simulink model "lss_online"  (R2022b)
settings: Solver=FixedStepAuto  StartTime=0.0  StopTime=Inf  FixedStep=0.001  RelTol=1e-3  EnableMultiTasking=on
InitFcn:
  | clear mex
model workspace (MAT data in the model file):
  worldsim_instance.endpoint_ip = '127.0.0.1'
  worldsim_instance.endpoint_port = 8080
values from neighbouring files (symbols this model uses):
  ADAS_Control_Mode = 1    [LSS_parameters.m]    (also in lss_ini_param.sldd = 1.0)
  AP_Transition_Rate = 0.5    [LSS_parameters.m]    (also in lss_ini_param.sldd = 0.8)
  butter_a = 1.0 -1.9911142922016536 0.99115359586893548    [lss_ini_param.sldd]
  butter_a_lka_out = 1.0 -1.5610180758007179 0.641351538057563    [lss_ini_param.sldd]
  butter_b = 9.825916820482009E-6 1.9651833640964018E-5 9.825916820482009E-6    [lss_ini_param.sldd]
  butter_b_lka_out = 0.020083365564211246 0.040166731128422492 0.020083365564211246    [lss_ini_param.sldd]
  index_variant_approaching_speed = 3.0    [lss_ini_param.sldd]
  LDW_Activity_Flag = 1    [LSS_parameters.m]    (also in lss_ini_param.sldd = 1.0)
  LDW_Freq_Hz = Sensor_Freq_worldsim    [LSS_parameters.m]    (also in lss_ini_param.sldd = 50.0)
  LDW_LaneGap_dydt_Warning = 50    [LSS_parameters.m]    (also in lss_ini_param.sldd = 50.0)
  LDW_LaneGap_Warning = [0.5 0.25]    [LSS_parameters.m]    (also in lss_ini_param.sldd = 0.5 0.25)
  LDW_Min_Speed = 60    [LSS_parameters.m]    (also in lss_ini_param.sldd = 60.0)
  LDW_Steer_Vibration_Amplitude = 5    [LSS_parameters.m]    (also in lss_ini_param.sldd = 5.0)
  LDW_Steer_Vibration_Freq = 25    [LSS_parameters.m]    (also in lss_ini_param.sldd = 25.0)
  LKA_Activity_Flag = 1    [LSS_parameters.m]    (also in lss_ini_param.sldd = 1.0)
  LKA_D = [0.2 0.3]    [LSS_parameters.m]    (also in lss_ini_param.sldd = 0.2 0.3)
  LKA_Dyn_Rate_Limiter_Gain = 0.1    [LSS_parameters.m]    (also in lss_ini_param.sldd)
  LKA_Dyn_Rate_Limiter_Power = 10    [LSS_parameters.m]    (also in lss_ini_param.sldd = 10.0)
  LKA_Error_dydt_Off = 1    [LSS_parameters.m]    (also in lss_ini_param.sldd = 1.0)
  LKA_Error_Max = 3    [LSS_parameters.m]    (also in lss_ini_param.sldd = 3.0)
  LKA_Error_Off = 0.5    [LSS_parameters.m]    (also in lss_ini_param.sldd)
  LKA_Freq_Hz = Sensor_Freq_worldsim    [LSS_parameters.m]    (also in lss_ini_param.sldd = 50.0)
  LKA_I = [0.025 0.05]    [LSS_parameters.m]    (also in lss_ini_param.sldd = 0.025 0.05)
  LKA_Lane_Gap_Activate = [0.25 0.125]    [LSS_parameters.m]    (also in lss_ini_param.sldd = -0.05 0.125)
  LKA_Lane_Gap_dydt_Activate = 50    [LSS_parameters.m]    (also in lss_ini_param.sldd = 50.0)
  LKA_Min_Speed = 60    [LSS_parameters.m]    (also in lss_ini_param.mat = 50; lss_ini_param.sldd = 50.0)
  LKA_On_Display_Freq = 5    [LSS_parameters.m]    (also in lss_ini_param.sldd = 5.0)
  LKA_P = [0.1 0.2]    [LSS_parameters.m]    (also in lss_ini_param.sldd = 0.1 0.2)
  LKA_Steer_Rate_Max_radps = 1    [LSS_parameters.m]    (also in lss_ini_param.sldd = 1.0)
  radar_source = 2    [LSS_parameters.m]    (also in lss_ini_param.sldd = 2.0)
  Sensor_Freq_worldsim = 50    [launcher.m]    (also in lss_ini_param.sldd = 50.0)
  target_speed = 72    [LSS_parameters.m]    (also in launcher.m = initCond.initialVelocity * 3.6)
  variant_approaching_speed = v_lat    [launcher.m]    (also in lss_ini_param.sldd = 0.2 0.3 0.4 0.5 0.6)
  vehicle_width = 1.86    [LSS_parameters.m]    (also in lss_ini_param.sldd = 2.05)
libraries: simulink x41, simwbSfunlib x40, slpidlib x3, viworldsim_lib x3
(part 1 of 2)
settings Model: DataDictionary=lss_ini_param.sldd  Creator=mcava  LastModifiedBy=pumpaipa
settings SolverCC: AlgebraicLoopSolver=TrustRegion  AutoInsertRateTranBlk=on
settings DataIOCC: LimitDataPoints=on  SaveFormat=Array  ReturnWorkspaceOutputs=off  SignalLoggingName=sigsOut
settings OptimizationCC: ExpressionDepthLimit=2147483647  InitFltsAndDblsToZero=on
settings DebuggingCC: SignalInfNanChecking=warning  UnderspecifiedInitializationDetection=Classic  MergeDetectMultiDrivingBlocksExec=none  SignalResolutionControl=TryResolveAllWithWarning  MultiTaskDSMMsg=warning  MultiTaskCondExecSysMsg=none  FcnCallInpInsideContextMsg=warning  UnconnectedInputMsg=warning  UnconnectedOutputMsg=warning  UnconnectedLineMsg=warning  StateNameClashWarn=warning  SFUnexpectedBacktrackingDiag=warning  SFNoUnconditionalDefaultTransitionDiag=warning  SFExecutionAtInitializationDiag=none  SFMachineParentedDataDiag=warning  ArithmeticOperatorsInVariantConditions=warning
settings HardwareCC: ProdBitPerLong=64  ProdHWDeviceType=Intel->x86-64 (Linux 64)  TargetHWDeviceType=32-bit Generic  TargetUnknown=on  ProdEqTarget=off
settings ModelReferenceCC: EnableRefExpFcnMdlSchedulingChecks=on  PropagateSignalLabelsOutOfModel=off
settings SFSimCC: SimUseLocalCustomCode=off  CustomCodeUndefinedFunction=UseInterfaceOnly
settings RTWCC: Description=VI-CarRealTime Solver Plugin V1.0  SystemTargetFile=vicrt_plugin.tlc  TemplateMakefile=vicrt_plugin_vcx64.tmf  PostCodeGenCommand=if strcmp(get_param(bdroot,'TemplateMakefile'),'vicrt_plugin_ccur.tmf'),copyfile([matlabroot,filesep,'rtw',filesep,'c',filesep,'tools',filesep,'unixtools.mk'],'unixtools.mk'),if ~verLessThan('matlab','9.6'),set_param(bdroot,'MatFileLogging','off'),end,end  RTWUseLocalCustomCode=off
settings CodeAppCC: MaxIdLength=80  StateflowObjectComments=on
settings STFCustomTargetCC: ModelReferenceCompliant=off  CombineOutputUpdateFcns=on  MatFileLogging=on  SystemTargetFile=vicrt_plugin.tlc
settings GRTTargetCC: TargetLangStandard=C89/C90 (ANSI)  ModelReferenceCompliant=off  ParMdlRefBuildCompliant=off  CompOptLevelCompliant=off  ConcurrentExecutionCompliant=off  CPPClassGenCompliant=off  UseToolchainInfoCompliant=off  RTWCAPIParams=on
settings ConfigComp: CovMetricSettings=dw  CovSaveCumulativeToWorkspaceVar=on  CovSaveSingleToWorkspaceVar=on  CovExternalEMLEnable=off

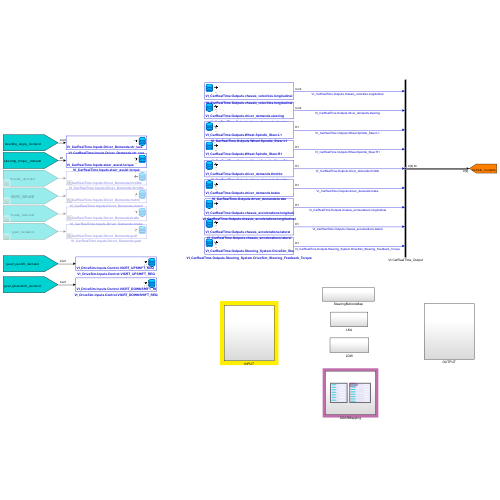
[thumbnail: Simulink's stored preview of the top-level diagram]
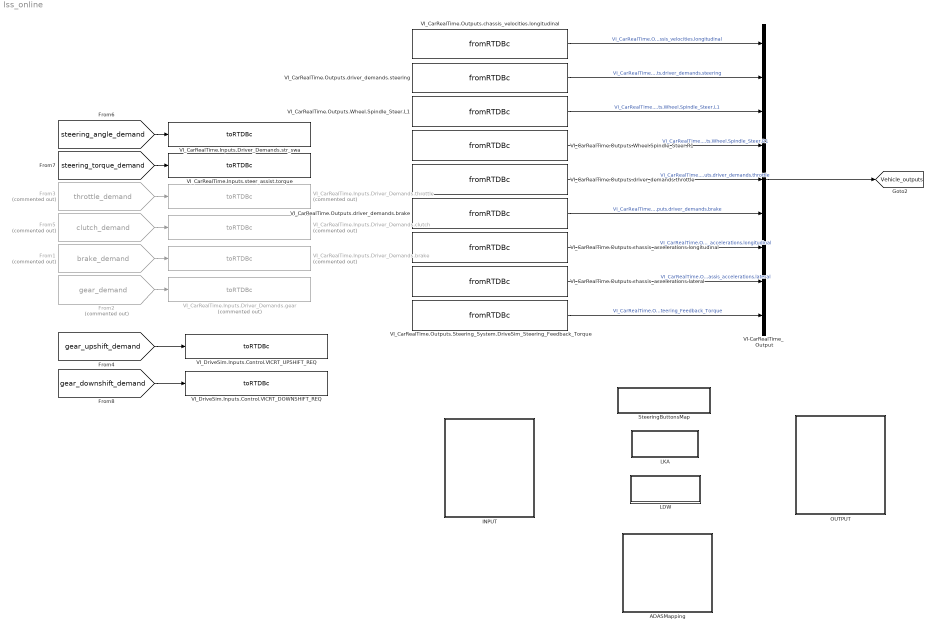
== system lss_online ==
  ADASMapping : Subsystem
  From1 : From  Commented=on  GotoTag=brake_demand  TagVisibility=global
  From2 : From  Commented=on  GotoTag=gear_demand  TagVisibility=global
  From3 : From  Commented=on  GotoTag=throttle_demand  TagVisibility=global
  From5 : From  Commented=on  GotoTag=clutch_demand  TagVisibility=global
  INPUT : Subsystem
  LDW : Subsystem
  LKA : Subsystem
  OUTPUT : Subsystem
  SteeringButtonsMap : Subsystem
  VI-CarRealTime_Output : BusCreator  Inputs=9
  VI_CarRealTime.Inputs.Driver_Demands.brake : simwbSfunlib/toRTDBc  Commented=on  stringBlock=off  varName=VI_CarRealTime.Inputs.Driver_Demands.brake  sigDim=[1 1]  sigType=double  sampleTime=[-1 0]  maxBuffSize=1024  busName=nobus  defaultValue=0  defaultString=simwbout  hasMapping=0  ptrName=VI_CarRealTime_Inputs_Driver_Demands_brake  enumOrAlias=nothing
      settings: SourceProductName=SimWB MLToolkit
  VI_CarRealTime.Inputs.Driver_Demands.clutch : simwbSfunlib/toRTDBc  Commented=on  stringBlock=off  varName=VI_CarRealTime.Inputs.Driver_Demands.clutch  sigDim=[1 1]  sigType=double  sampleTime=[-1 0]  maxBuffSize=1024  busName=nobus  defaultValue=0  defaultString=simwbout  hasMapping=0  ptrName=VI_CarRealTime_Inputs_Driver_Demands_clutch  enumOrAlias=nothing
      settings: SourceProductName=SimWB MLToolkit
  VI_CarRealTime.Inputs.Driver_Demands.gear : simwbSfunlib/toRTDBc  Commented=on  stringBlock=off  varName=VI_CarRealTime.Inputs.Driver_Demands.gear  sigDim=[1 1]  sigType=double  sampleTime=[-1 0]  maxBuffSize=1024  busName=nobus  defaultValue=0  defaultString=simwbout  hasMapping=0  ptrName=VI_CarRealTime_Inputs_Driver_Demands_gear  enumOrAlias=nothing
      settings: SourceProductName=SimWB MLToolkit
  VI_CarRealTime.Inputs.Driver_Demands.str_swa : simwbSfunlib/toRTDBc  stringBlock=off  varName=VI_CarRealTime.Inputs.Driver_Demands.str_swa  sigDim=[1 1]  sigType=double  sampleTime=[-1 0]  maxBuffSize=1024  busName=nobus  defaultValue=0  defaultString=simwbout  hasMapping=0  ptrName=VI_CarRealTime_Inputs_Driver_Demands_str_swa  enumOrAlias=nothing
      settings: SourceProductName=SimWB MLToolkit
  VI_CarRealTime.Inputs.Driver_Demands.throttle : simwbSfunlib/toRTDBc  Commented=on  stringBlock=off  varName=VI_CarRealTime.Inputs.Driver_Demands.throttle  sigDim=[1 1]  sigType=double  sampleTime=[-1 0]  maxBuffSize=1024  busName=nobus  defaultValue=0  defaultString=simwbout  hasMapping=0  ptrName=VI_CarRealTime_Inputs_Driver_Demands_throttle  enumOrAlias=nothing
      settings: SourceProductName=SimWB MLToolkit
  VI_CarRealTime.Inputs.steer_assist.torque : simwbSfunlib/toRTDBc  stringBlock=off  varName=VI_CarRealTime.Inputs.steer_assist.torque  sigDim=[1 1]  sigType=double  sampleTime=[-1 0]  maxBuffSize=1024  busName=nobus  defaultValue=0  defaultString=simwbout  hasMapping=0  ptrName=VI_CarRealTime_Inputs_steer_assist_torque  enumOrAlias=nothing
      settings: SourceProductName=SimWB MLToolkit
  VI_CarRealTime.Outputs.Steering_System.DriveSim_Steering_Feedback_Torque : simwbSfunlib/fromRTDBc  stringBlock=off  varName=VI_CarRealTime.Outputs.Steering_System.DriveSim_Steering_Feedback_Torque  sigDim=[1 1]  sigType=double  sampleTime=[-1 0]  maxBuffSize=1024  busName=nobus  defaultValue=0  defaultString=simwbin  hasMapping=0  ptrName=VI_CarRealTime_Outputs_Steering_System_DriveSim_Steering_Feedback_Torque  enumOrAlias=nothing
      settings: SourceProductName=SimWB MLToolkit
  VI_CarRealTime.Outputs.Wheel.Spindle_Steer.L1 : simwbSfunlib/fromRTDBc  stringBlock=off  varName=VI_CarRealTime.Outputs.Wheel.Spindle_Steer.L1  sigDim=[1 1]  sigType=double  sampleTime=[-1 0]  maxBuffSize=1024  busName=nobus  defaultValue=0  defaultString=simwbin  hasMapping=0  ptrName=VI_CarRealTime_Outputs_Wheel_Spindle_Steer_L1  enumOrAlias=nothing
      settings: SourceProductName=SimWB MLToolkit
  VI_CarRealTime.Outputs.Wheel.Spindle_Steer.R1 : simwbSfunlib/fromRTDBc  stringBlock=off  varName=VI_CarRealTime.Outputs.Wheel.Spindle_Steer.R1  sigDim=[1 1]  sigType=double  sampleTime=[-1 0]  maxBuffSize=1024  busName=nobus  defaultValue=0  defaultString=simwbin  hasMapping=0  ptrName=VI_CarRealTime_Outputs_Wheel_Spindle_Steer_R1  enumOrAlias=nothing
      settings: SourceProductName=SimWB MLToolkit
  VI_CarRealTime.Outputs.chassis_accelerations.lateral : simwbSfunlib/fromRTDBc  stringBlock=off  varName=VI_CarRealTime.Outputs.chassis_accelerations.lateral  sigDim=[1 1]  sigType=double  sampleTime=[-1 0]  maxBuffSize=1024  busName=nobus  defaultValue=0  defaultString=simwbin  hasMapping=0  ptrName=VI_CarRealTime_Outputs_chassis_accelerations_lateral  enumOrAlias=nothing
      settings: SourceProductName=SimWB MLToolkit
  VI_CarRealTime.Outputs.chassis_accelerations.longitudinal : simwbSfunlib/fromRTDBc  stringBlock=off  varName=VI_CarRealTime.Outputs.chassis_accelerations.longitudinal  sigDim=[1 1]  sigType=double  sampleTime=[-1 0]  maxBuffSize=1024  busName=nobus  defaultValue=0  defaultString=simwbin  hasMapping=0  ptrName=VI_CarRealTime_Outputs_chassis_accelerations_longitudinal  enumOrAlias=nothing
      settings: SourceProductName=SimWB MLToolkit
  VI_CarRealTime.Outputs.chassis_velocities.longitudinal : simwbSfunlib/fromRTDBc  stringBlock=off  varName=VI_CarRealTime.Outputs.chassis_velocities.longitudinal  sigDim=[1 1]  sigType=double  sampleTime=[-1 0]  maxBuffSize=1024  busName=nobus  defaultValue=0  defaultString=simwbin  hasMapping=0  ptrName=VI_CarRealTime_Outputs_chassis_velocities_longitudinal  enumOrAlias=nothing
      settings: SourceProductName=SimWB MLToolkit
  VI_CarRealTime.Outputs.driver_demands.brake : simwbSfunlib/fromRTDBc  stringBlock=off  varName=VI_CarRealTime.Outputs.driver_demands.brake  sigDim=[1 1]  sigType=double  sampleTime=[-1 0]  maxBuffSize=1024  busName=nobus  defaultValue=0  defaultString=simwbin  hasMapping=0  ptrName=VI_CarRealTime_Outputs_driver_demands_brake  enumOrAlias=nothing
      settings: SourceProductName=SimWB MLToolkit
  VI_CarRealTime.Outputs.driver_demands.steering : simwbSfunlib/fromRTDBc  stringBlock=off  varName=VI_CarRealTime.Outputs.driver_demands.steering  sigDim=[1 1]  sigType=double  sampleTime=[-1 0]  maxBuffSize=1024  busName=nobus  defaultValue=0  defaultString=simwbin  hasMapping=0  ptrName=VI_CarRealTime_Outputs_driver_demands_steering  enumOrAlias=nothing
      settings: SourceProductName=SimWB MLToolkit
  VI_CarRealTime.Outputs.driver_demands.throttle : simwbSfunlib/fromRTDBc  stringBlock=off  varName=VI_CarRealTime.Outputs.driver_demands.throttle  sigDim=[1 1]  sigType=double  sampleTime=[-1 0]  maxBuffSize=1024  busName=nobus  defaultValue=0  defaultString=simwbin  hasMapping=0  ptrName=VI_CarRealTime_Outputs_driver_demands_throttle  enumOrAlias=nothing
      settings: SourceProductName=SimWB MLToolkit
  VI_DriveSim.Inputs.Control.VICRT_DOWNSHIFT_REQ : simwbSfunlib/toRTDBc  stringBlock=off  varName=VI_DriveSim.Inputs.Control.VICRT_DOWNSHIFT_REQ  sigDim=[1 1]  sigType=double  sampleTime=[-1 0]  maxBuffSize=1024  busName=nobus  defaultValue=0  defaultString=simwbout  hasMapping=0  ptrName=VI_DriveSim_Inputs_Control_VICRT_DOWNSHIFT_REQ  enumOrAlias=nothing
      settings: SourceProductName=SimWB MLToolkit
  VI_DriveSim.Inputs.Control.VICRT_UPSHIFT_REQ : simwbSfunlib/toRTDBc  stringBlock=off  varName=VI_DriveSim.Inputs.Control.VICRT_UPSHIFT_REQ  sigDim=[1 1]  sigType=double  sampleTime=[-1 0]  maxBuffSize=1024  busName=nobus  defaultValue=0  defaultString=simwbout  hasMapping=0  ptrName=VI_DriveSim_Inputs_Control_VICRT_UPSHIFT_REQ  enumOrAlias=nothing
      settings: SourceProductName=SimWB MLToolkit
  tag scope: Vehicle_outputs=global
  wires:
  VI-CarRealTime_Output/1 -> [Vehicle_outputs]
  [steering_angle_demand] -> VI_CarRealTime.Inputs.Driver_Demands.str_swa/1
  [steering_torque_demand] -> VI_CarRealTime.Inputs.steer_assist.torque/1
  From3/1 -> VI_CarRealTime.Inputs.Driver_Demands.throttle/1
  From5/1 -> VI_CarRealTime.Inputs.Driver_Demands.clutch/1
  From1/1 -> VI_CarRealTime.Inputs.Driver_Demands.brake/1
  From2/1 -> VI_CarRealTime.Inputs.Driver_Demands.gear/1
  VI_CarRealTime.Outputs.Wheel.Spindle_Steer.R1/1 -> VI-CarRealTime_Output/4  "VI_CarRealTime.Outputs.Wheel.Spindle_Steer.R1"
  VI_CarRealTime.Outputs.chassis_velocities.longitudinal/1 -> VI-CarRealTime_Output/1  "VI_CarRealTime.Outputs.chassis_velocities.longitudinal"
  VI_CarRealTime.Outputs.Steering_System.DriveSim_Steering_Feedback_Torque/1 -> VI-CarRealTime_Output/9  "VI_CarRealTime.Outputs.Steering_System.DriveSim_Steering_Feedback_Torque"
  VI_CarRealTime.Outputs.chassis_accelerations.lateral/1 -> VI-CarRealTime_Output/8  "VI_CarRealTime.Outputs.chassis_accelerations.lateral"
  VI_CarRealTime.Outputs.driver_demands.brake/1 -> VI-CarRealTime_Output/6  "VI_CarRealTime.Outputs.driver_demands.brake"
  VI_CarRealTime.Outputs.Wheel.Spindle_Steer.L1/1 -> VI-CarRealTime_Output/3  "VI_CarRealTime.Outputs.Wheel.Spindle_Steer.L1"
  VI_CarRealTime.Outputs.driver_demands.throttle/1 -> VI-CarRealTime_Output/5  "VI_CarRealTime.Outputs.driver_demands.throttle"
  VI_CarRealTime.Outputs.driver_demands.steering/1 -> VI-CarRealTime_Output/2  "VI_CarRealTime.Outputs.driver_demands.steering"
  VI_CarRealTime.Outputs.chassis_accelerations.longitudinal/1 -> VI-CarRealTime_Output/7  "VI_CarRealTime.Outputs.chassis_accelerations.longitudinal"
  [gear_upshift_demand] -> VI_DriveSim.Inputs.Control.VICRT_UPSHIFT_REQ/1
  [gear_downshift_demand] -> VI_DriveSim.Inputs.Control.VICRT_DOWNSHIFT_REQ/1

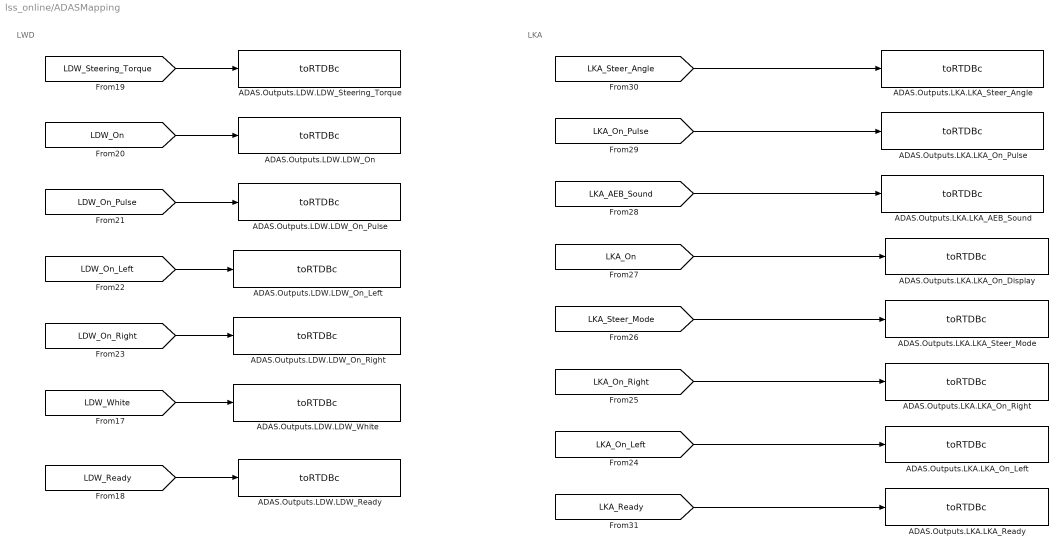
== system lss_online/ADASMapping ==
  note: LKA
  note: LWD
  ADAS.Outputs.LDW.LDW_On : simwbSfunlib/toRTDBc  stringBlock=off  varName=ADAS.Outputs.LDW.LDW_On  sigDim=[1 1]  sigType=double  sampleTime=[-1 0]  maxBuffSize=1024  busName=nobus  defaultValue=0  defaultString=simwbout  hasMapping=0  ptrName=ADAS_Outputs_LDW_LDW_On  enumOrAlias=nothing
      settings: SourceProductName=SimWB MLToolkit
  ADAS.Outputs.LDW.LDW_On_Left : simwbSfunlib/toRTDBc  stringBlock=off  varName=ADAS.Outputs.LDW.LDW_On_Left  sigDim=[1 1]  sigType=double  sampleTime=[-1 0]  maxBuffSize=1024  busName=nobus  defaultValue=0  defaultString=simwbout  hasMapping=0  ptrName=ADAS_Outputs_LDW_LDW_On_Left  enumOrAlias=nothing
      settings: SourceProductName=SimWB MLToolkit
  ADAS.Outputs.LDW.LDW_On_Pulse : simwbSfunlib/toRTDBc  stringBlock=off  varName=ADAS.Outputs.LDW.LDW_On_Pulse  sigDim=[1 1]  sigType=double  sampleTime=[-1 0]  maxBuffSize=1024  busName=nobus  defaultValue=0  defaultString=simwbout  hasMapping=0  ptrName=ADAS_Outputs_LDW_LDW_On_Pulse  enumOrAlias=nothing
      settings: SourceProductName=SimWB MLToolkit
  ADAS.Outputs.LDW.LDW_On_Right : simwbSfunlib/toRTDBc  stringBlock=off  varName=ADAS.Outputs.LDW.LDW_On_Right  sigDim=[1 1]  sigType=double  sampleTime=[-1 0]  maxBuffSize=1024  busName=nobus  defaultValue=0  defaultString=simwbout  hasMapping=0  ptrName=ADAS_Outputs_LDW_LDW_On_Right  enumOrAlias=nothing
      settings: SourceProductName=SimWB MLToolkit
  ADAS.Outputs.LDW.LDW_Ready : simwbSfunlib/toRTDBc  stringBlock=off  varName=ADAS.Outputs.LDW.LDW_Ready  sigDim=[1 1]  sigType=double  sampleTime=[-1 0]  maxBuffSize=1024  busName=nobus  defaultValue=0  defaultString=simwbout  hasMapping=0  ptrName=ADAS_Outputs_LDW_LDW_Ready  enumOrAlias=nothing
      settings: SourceProductName=SimWB MLToolkit
  ADAS.Outputs.LDW.LDW_Steering_Torque : simwbSfunlib/toRTDBc  stringBlock=off  varName=ADAS.Outputs.LDW.LDW_Steering_Torque  sigDim=[1 1]  sigType=double  sampleTime=[-1 0]  maxBuffSize=1024  busName=nobus  defaultValue=0  defaultString=simwbout  hasMapping=0  ptrName=ADAS_Outputs_LDW_LDW_Steering_Torque  enumOrAlias=nothing
      settings: SourceProductName=SimWB MLToolkit
  ADAS.Outputs.LDW.LDW_White : simwbSfunlib/toRTDBc  stringBlock=off  varName=ADAS.Outputs.LDW.LDW_White  sigDim=[1 1]  sigType=double  sampleTime=[-1 0]  maxBuffSize=1024  busName=nobus  defaultValue=0  defaultString=simwbout  hasMapping=0  ptrName=ADAS_Outputs_LDW_LDW_White  enumOrAlias=nothing
      settings: SourceProductName=SimWB MLToolkit
  ADAS.Outputs.LKA.LKA_AEB_Sound : simwbSfunlib/toRTDBc  stringBlock=off  varName=ADAS.Outputs.LKA.LKA_AEB_Sound  sigDim=[1 1]  sigType=double  sampleTime=[-1 0]  maxBuffSize=1024  busName=nobus  defaultValue=0  defaultString=simwbout  hasMapping=0  ptrName=ADAS_Outputs_LKA_LKA_AEB_Sound  enumOrAlias=nothing
      settings: SourceProductName=SimWB MLToolkit
  ADAS.Outputs.LKA.LKA_On_Display : simwbSfunlib/toRTDBc  stringBlock=off  varName=ADAS.Outputs.LKA.LKA_On_Display  sigDim=[1 1]  sigType=double  sampleTime=[-1 0]  maxBuffSize=1024  busName=nobus  defaultValue=0  defaultString=simwbout  hasMapping=0  ptrName=ADAS_Outputs_LKA_LKA_On_Display  enumOrAlias=nothing
      settings: SourceProductName=SimWB MLToolkit
  ADAS.Outputs.LKA.LKA_On_Left : simwbSfunlib/toRTDBc  stringBlock=off  varName=ADAS.Outputs.LKA.LKA_On_Left  sigDim=[1 1]  sigType=double  sampleTime=[-1 0]  maxBuffSize=1024  busName=nobus  defaultValue=0  defaultString=simwbout  hasMapping=0  ptrName=ADAS_Outputs_LKA_LKA_On_Left  enumOrAlias=nothing
      settings: SourceProductName=SimWB MLToolkit
  ADAS.Outputs.LKA.LKA_On_Pulse : simwbSfunlib/toRTDBc  stringBlock=off  varName=ADAS.Outputs.LKA.LKA_On_Pulse  sigDim=[1 1]  sigType=double  sampleTime=[-1 0]  maxBuffSize=1024  busName=nobus  defaultValue=0  defaultString=simwbout  hasMapping=0  ptrName=ADAS_Outputs_LKA_LKA_On_Pulse  enumOrAlias=nothing
      settings: SourceProductName=SimWB MLToolkit
  ADAS.Outputs.LKA.LKA_On_Right : simwbSfunlib/toRTDBc  stringBlock=off  varName=ADAS.Outputs.LKA.LKA_On_Right  sigDim=[1 1]  sigType=double  sampleTime=[-1 0]  maxBuffSize=1024  busName=nobus  defaultValue=0  defaultString=simwbout  hasMapping=0  ptrName=ADAS_Outputs_LKA_LKA_On_Right  enumOrAlias=nothing
      settings: SourceProductName=SimWB MLToolkit
  ADAS.Outputs.LKA.LKA_Ready : simwbSfunlib/toRTDBc  stringBlock=off  varName=ADAS.Outputs.LKA.LKA_Ready  sigDim=[1 1]  sigType=double  sampleTime=[-1 0]  maxBuffSize=1024  busName=nobus  defaultValue=0  defaultString=simwbout  hasMapping=0  ptrName=ADAS_Outputs_LKA_LKA_Ready  enumOrAlias=nothing
      settings: SourceProductName=SimWB MLToolkit
  ADAS.Outputs.LKA.LKA_Steer_Angle : simwbSfunlib/toRTDBc  stringBlock=off  varName=ADAS.Outputs.LKA.LKA_Steer_Angle  sigDim=[1 1]  sigType=double  sampleTime=[-1 0]  maxBuffSize=1024  busName=nobus  defaultValue=0  defaultString=simwbout  hasMapping=0  ptrName=ADAS_Outputs_LKA_LKA_Steer_Angle  enumOrAlias=nothing
      settings: SourceProductName=SimWB MLToolkit
  ADAS.Outputs.LKA.LKA_Steer_Mode : simwbSfunlib/toRTDBc  stringBlock=off  varName=ADAS.Outputs.LKA.LKA_Steer_Mode  sigDim=[1 1]  sigType=double  sampleTime=[-1 0]  maxBuffSize=1024  busName=nobus  defaultValue=0  defaultString=simwbout  hasMapping=0  ptrName=ADAS_Outputs_LKA_LKA_Steer_Mode  enumOrAlias=nothing
      settings: SourceProductName=SimWB MLToolkit
  wires:
  [LKA_On_Right] -> ADAS.Outputs.LKA.LKA_On_Right/1
  [LKA_On] -> ADAS.Outputs.LKA.LKA_On_Display/1
  [LKA_On_Pulse] -> ADAS.Outputs.LKA.LKA_On_Pulse/1
  [LKA_Steer_Angle] -> ADAS.Outputs.LKA.LKA_Steer_Angle/1
  [LKA_On_Left] -> ADAS.Outputs.LKA.LKA_On_Left/1
  [LKA_Ready] -> ADAS.Outputs.LKA.LKA_Ready/1
  [LKA_AEB_Sound] -> ADAS.Outputs.LKA.LKA_AEB_Sound/1
  [LKA_Steer_Mode] -> ADAS.Outputs.LKA.LKA_Steer_Mode/1
  [LDW_Steering_Torque] -> ADAS.Outputs.LDW.LDW_Steering_Torque/1
  [LDW_On] -> ADAS.Outputs.LDW.LDW_On/1
  [LDW_On_Pulse] -> ADAS.Outputs.LDW.LDW_On_Pulse/1
  [LDW_Ready] -> ADAS.Outputs.LDW.LDW_Ready/1
  [LDW_On_Right] -> ADAS.Outputs.LDW.LDW_On_Right/1
  [LDW_On_Left] -> ADAS.Outputs.LDW.LDW_On_Left/1
  [LDW_White] -> ADAS.Outputs.LDW.LDW_White/1

== system lss_online/INPUT ==
  Inputs for CRT : Subsystem
  finalizing controls inputs : Subsystem
  simple_cruise_control : Subsystem  Commented=on

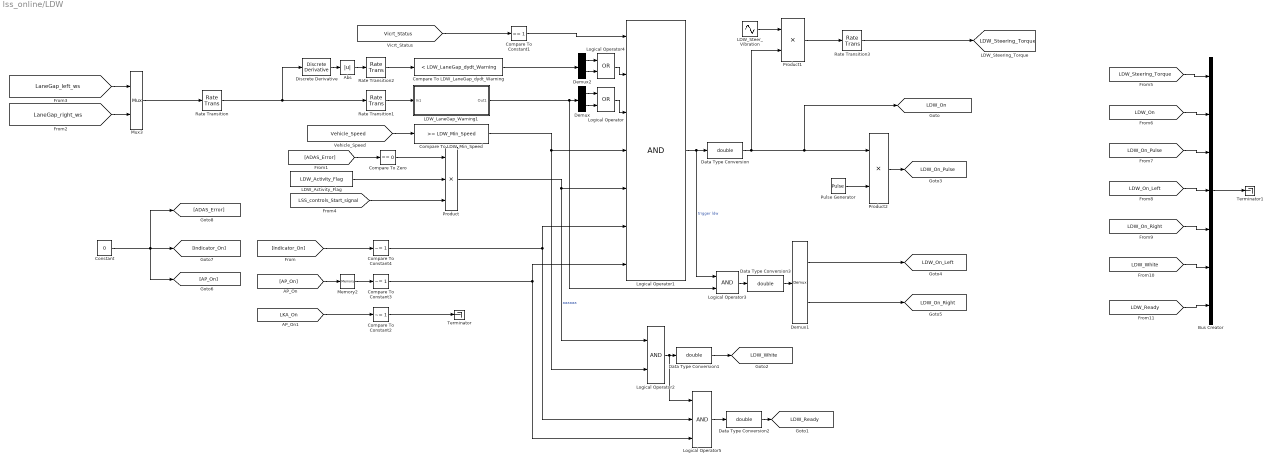
== system lss_online/LDW ==
  Abs : Abs  SaturateOnIntegerOverflow=off
  Bus Creator : BusCreator  Inputs=7
  Compare To Constant1 : simulink/Logic and Bit Operations/Compare To Constant  relop===  const=1  OutDataTypeStr=boolean
  Compare To Constant2 : simulink/Logic and Bit Operations/Compare To Constant  relop=~=  const=1  OutDataTypeStr=boolean
  Compare To Constant3 : simulink/Logic and Bit Operations/Compare To Constant  relop=~=  const=1  OutDataTypeStr=boolean
  Compare To Constant4 : simulink/Logic and Bit Operations/Compare To Constant  relop=~=  const=1  OutDataTypeStr=boolean
  Compare To Zero : simulink/Logic and Bit Operations/Compare To Zero  relop===  OutDataTypeStr=boolean
  Compare To LDW_LaneGap_dydt_Warning : simulink/Logic and Bit Operations/Compare To Constant  relop=<  const=LDW_LaneGap_dydt_Warning  OutDataTypeStr=boolean
  Compare To LDW_Min_Speed : simulink/Logic and Bit Operations/Compare To Constant  relop=>=  const=LDW_Min_Speed  OutDataTypeStr=boolean
  Constant : Constant  Value=0
  Data Type Conversion{,1..3} (4 alike) : DataTypeConversion  OutDataTypeStr=double  SaturateOnIntegerOverflow=off  RndMeth=Floor
  Demux : Demux  Outputs=2
  Demux1 : Demux  Outputs=2
  Demux2 : Demux  Outputs=2
  Discrete Derivative : simulink/Discrete/Discrete Derivative  gainval=1.0  ICPrevScaledInput=0.0  OutMin=[]  OutMax=[]  OutDataType=fixdt(1, 16)  OutScaling=2^-10  DoSatur=off
  LDW_Activity_Flag : Constant  Value=LDW_Activity_Flag
  LDW_LaneGap_Warning1 : Subsystem
  LDW_Steer_Vibration : Sin  Amplitude=LDW_Steer_Vibration_Amplitude  Frequency=LDW_Steer_Vibration_Freq*2*pi  SampleTime=0
  Logical Operator : Logic  Operator=OR  AllPortsSameDT=off  OutDataTypeStr=boolean
  Logical Operator1 : Logic  Inputs=7  AllPortsSameDT=off  OutDataTypeStr=boolean
  Logical Operator2 : Logic  AllPortsSameDT=off  OutDataTypeStr=boolean
  Logical Operator3 : Logic  AllPortsSameDT=off  OutDataTypeStr=boolean
  Logical Operator4 : Logic  Operator=OR  AllPortsSameDT=off  OutDataTypeStr=boolean
  Logical Operator5 : Logic  Inputs=3  AllPortsSameDT=off  OutDataTypeStr=boolean
  Memory2 : Memory
  Mux3 : Mux  Inputs=2
  Product : Product  Inputs=3
  Product1 : Product
  Product2 : Product
  Pulse Generator : DiscretePulseGenerator  PulseType=Time based  Period=1/LKA_On_Display_Freq  PulseWidth=50
  Rate Transition : RateTransition  OutPortSampleTime=1/LDW_Freq_Hz
  Rate Transition1 : RateTransition  OutPortSampleTime=1/1000
  Rate Transition2 : RateTransition  OutPortSampleTime=1/1000
  Rate Transition3 : RateTransition  OutPortSampleTime=1/1000
  Terminator : Terminator
  Terminator1 : Terminator
  tag scope: LDW_On=global, LDW_On_Left=global, LDW_On_Pulse=global, LDW_On_Right=global, LDW_Ready=global, LDW_Steering_Torque=global, LDW_White=global
  wires:
  [Vicrt_Status] -> Compare To Constant1/1
  Compare To Constant1/1 -> Logical Operator1/1
  Logical Operator1/1 -> Logical Operator3/1, Data Type Conversion/1  "trigger ldw"
  [Vehicle_Speed] -> Compare To LDW_Min_Speed/1
  Compare To LDW_Min_Speed/1 -> Logical Operator2/2, Logical Operator1/4
  Logical Operator/1 -> Logical Operator1/3
  LDW_Steer_Vibration/1 -> Product1/1
  Product1/1 -> Rate Transition3/1
  Data Type Conversion/1 -> Product2/1, [LDW_On], Product1/2
  Logical Operator2/1 -> Logical Operator5/1, Data Type Conversion1/1
  Data Type Conversion1/1 -> [LDW_White]
  Demux/1 -> Logical Operator/1
  Demux/2 -> Logical Operator/2
  Demux1/1 -> [LDW_On_Left]
  Demux1/2 -> [LDW_On_Right]
  Data Type Conversion3/1 -> Demux1/1
  Logical Operator3/1 -> Data Type Conversion3/1
  Rate Transition/1 -> Rate Transition1/1, Discrete Derivative/1
  Discrete Derivative/1 -> Abs/1
  Rate Transition2/1 -> Compare To LDW_LaneGap_dydt_Warning/1
  Compare To LDW_LaneGap_dydt_Warning/1 -> Demux2/1
  Logical Operator4/1 -> Logical Operator1/2
  Demux2/1 -> Logical Operator4/1
  Demux2/2 -> Logical Operator4/2
  Abs/1 -> Rate Transition2/1
  [Indicator_On] -> Compare To Constant4/1
  Compare To Constant4/1 -> Logical Operator1/6, Logical Operator5/2
  Logical Operator5/1 -> Data Type Conversion2/1
  Product/1 -> Logical Operator2/1, Logical Operator1/5  "aaaaaa"
  [ADAS_Error] -> Compare To Zero/1
  Compare To Zero/1 -> Product/1
  LDW_Activity_Flag/1 -> Product/2
  LDW_LaneGap_Warning1/1(Out1) -> Logical Operator3/2, Demux/1
  Rate Transition1/1 -> LDW_LaneGap_Warning1/1(In1)
  [AP_On] -> Memory2/1
  Memory2/1 -> Compare To Constant3/1
  Compare To Constant3/1 -> Logical Operator1/7, Logical Operator5/3
  Pulse Generator/1 -> Product2/2
  Product2/1 -> [LDW_On_Pulse]
  [LKA_On] -> Compare To Constant2/1
  Compare To Constant2/1 -> Terminator/1
  Rate Transition3/1 -> [LDW_Steering_Torque]
  Data Type Conversion2/1 -> [LDW_Ready]
  Mux3/1 -> Rate Transition/1
  [LaneGap_left_ws] -> Mux3/1
  [LaneGap_right_ws] -> Mux3/2
  [LSS_controls_Start_signal] -> Product/3
  Constant/1 -> [AP_On], [ADAS_Error], [Indicator_On]
  [LDW_Steering_Torque] -> Bus Creator/1
  [LDW_On] -> Bus Creator/2
  [LDW_On_Pulse] -> Bus Creator/3
  [LDW_On_Left] -> Bus Creator/4
  [LDW_On_Right] -> Bus Creator/5
  [LDW_White] -> Bus Creator/6
  [LDW_Ready] -> Bus Creator/7
  Bus Creator/1 -> Terminator1/1

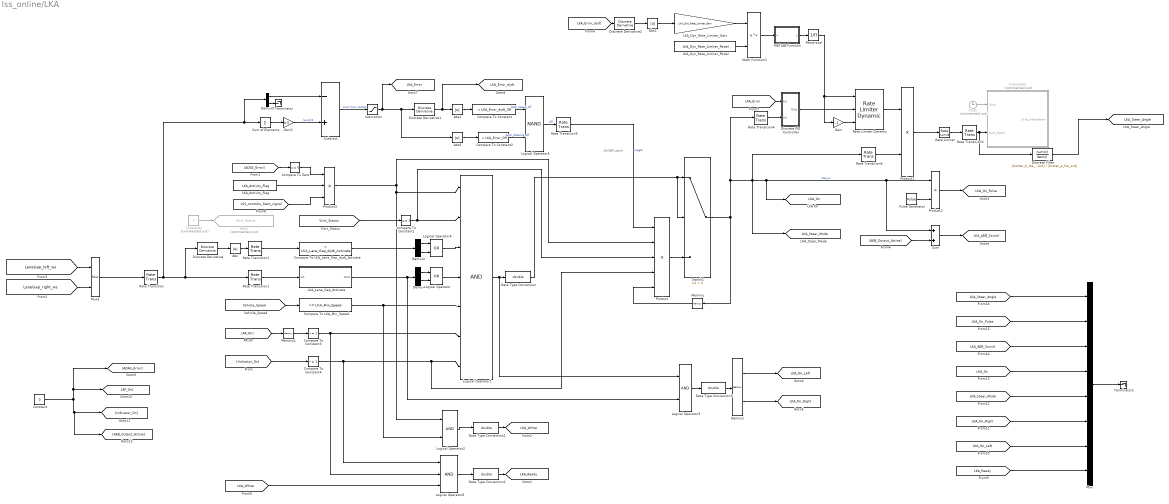
== system lss_online/LKA ==
  note: On/Off Latch
  Abs{,1..3} (4 alike) : Abs  SaturateOnIntegerOverflow=off
  Clock : Clock  Commented=on
  Compare To Constant : simulink/Logic and Bit Operations/Compare To Constant  relop=<  const=LKA_Error_dydt_Off  OutDataTypeStr=boolean
  Compare To Constant1 : simulink/Logic and Bit Operations/Compare To Constant  relop===  const=1  OutDataTypeStr=boolean
  Compare To Constant2 : simulink/Logic and Bit Operations/Compare To Constant  relop=<  const=LKA_Error_Off  OutDataTypeStr=boolean
  Compare To Constant3 : simulink/Logic and Bit Operations/Compare To Constant  relop=~=  const=1  OutDataTypeStr=boolean
  Compare To Constant4 : simulink/Logic and Bit Operations/Compare To Constant  relop=~=  const=1  OutDataTypeStr=boolean
  Compare To LKA_Lane_Gap_dydt_Activate : simulink/Logic and Bit Operations/Compare To Constant  relop=<  const=LKA_Lane_Gap_dydt_Activate  OutDataTypeStr=boolean
  Compare To LKA_Min_Speed : simulink/Logic and Bit Operations/Compare To Constant  relop=>=  const=LKA_Min_Speed  OutDataTypeStr=boolean
  Compare To Zero : simulink/Logic and Bit Operations/Compare To Zero  relop===  OutDataTypeStr=boolean
  Constant : Constant  Value=0
  Constant1 : Constant  Commented=on
  Data Type Conversion{,1..3} (4 alike) : DataTypeConversion  OutDataTypeStr=double  SaturateOnIntegerOverflow=off  RndMeth=Floor
  Demux{,1..3} (4 alike) : Demux  Outputs=2
  Discrete Derivative : simulink/Discrete/Discrete Derivative  gainval=1.0  ICPrevScaledInput=0.0  OutMin=[]  OutMax=[]  OutDataType=fixdt(1, 16)  OutScaling=2^-10  DoSatur=off
  Discrete Derivative1 : simulink/Discrete/Discrete Derivative  gainval=1.0  ICPrevScaledInput=0.0  OutMin=[]  OutMax=[]  OutDataType=fixdt(1, 16)  OutScaling=2^-10  DoSatur=off
  Discrete Derivative2 : simulink/Discrete/Discrete Derivative  gainval=1.0  ICPrevScaledInput=0.0  OutMin=[]  OutMax=[]  OutDataType=fixdt(1, 16)  OutScaling=2^-10  DoSatur=off
  Discrete Filter : DiscreteFilter  Numerator=[butter_b_lka_out]  Denominator=[butter_a_lka_out]  SampleTime=1e-3
  Discrete PID Controller : Subsystem
  Gain : Gain  Gain=-1
  Gain1 : Gain  Gain=0.5
  Goto : Goto  Commented=on  GotoTag=Vicrt_Status  TagVisibility=global
  LKA_Activity_Flag : Constant  Value=LKA_Activity_Flag
  LKA_Dyn_Rate_Limiter_Gain : Gain  Gain=LKA_Dyn_Rate_Limiter_Gain
  LKA_Dyn_Rate_Limiter_Power : Constant  Value=LKA_Dyn_Rate_Limiter_Power
  LKA_Lane_Gap_Activate : Subsystem
  Logical Operator : Logic  Operator=OR  AllPortsSameDT=off  OutDataTypeStr=boolean
  Logical Operator1 : Logic  Inputs=7  AllPortsSameDT=off  OutDataTypeStr=boolean
  Logical Operator2 : Logic  AllPortsSameDT=off  OutDataTypeStr=boolean
  Logical Operator3 : Logic  AllPortsSameDT=off  OutDataTypeStr=boolean
  Logical Operator4 : Logic  Operator=OR  AllPortsSameDT=off  OutDataTypeStr=boolean
  Logical Operator5 : Logic  Operator=NAND  AllPortsSameDT=off  OutDataTypeStr=boolean
  Logical Operator6 : Logic  Inputs=3  AllPortsSameDT=off  OutDataTypeStr=boolean
  MATLAB Function : MATLAB Function  TreatAsAtomicUnit=on
  Math Function1 : Math  Operator=pow  SignedPower=on
  Memory : Memory
  Memory2 : Memory
  Mux : Mux  Inputs=8
  Mux3 : Mux  Inputs=2
  Product : Product  Inputs=5
  Product1 : Product
  Product2 : Product
  Product3 : Product  Inputs=3
  Pulse Generator : DiscretePulseGenerator  PulseType=Time based  Period=1/LKA_On_Display_Freq  PulseWidth=50
  Rate Limiter : RateLimiter  RisingSlewLimit=LKA_Steer_Rate_Max_radps  FallingSlewLimit=-LKA_Steer_Rate_Max_radps  SampleTimeMode=inherited
  Rate Limiter Dynamic : simulink/Discontinuities/Rate Limiter Dynamic
  Rate Transition : RateTransition  OutPortSampleTime=1/LKA_Freq_Hz
  Rate Transition{1..3,5} (4 alike) : RateTransition  OutPortSampleTime=1/1000
  Rate Transition4 : RateTransition  OutPortSampleTime=1/LKA_Freq_Hz
  Rate Transition6 : RateTransition  OutPortSampleTime=1/LKA_Freq_Hz
  Reciprocal : Product  Inputs=/  RndMeth=Zero  SaturateOnIntegerOverflow=on
  Saturation : Saturate  UpperLimit=LKA_Error_Max  LowerLimit=-LKA_Error_Max
  Subsystem : Subsystem  Commented=on
  Subtract : Sum  Inputs=-+
  Sum : Sum
  Sum of Elements : Sum  Inputs=+
  Switch1 : Switch  Criteria=u2 > Threshold  SaturateOnIntegerOverflow=off  InputSameDT=off
  Terminator : Terminator
  Terminator1 : Terminator
  tag scope: LKA_AEB_Sound=global, LKA_Error=global, LKA_Error_dydt=global, LKA_On=global, LKA_On_Left=global, LKA_On_Pulse=global, LKA_On_Right=global, LKA_Ready=global, LKA_Steer_Angle=global, LKA_Steer_Mode=global, LKA_White=global
  wires:
  [Vicrt_Status] -> Compare To Constant1/1
  Compare To Constant1/1 -> Product/3, Logical Operator1/2
  Logical Operator1/1 -> Logical Operator3/1, Data Type Conversion/1
  [Vehicle_Speed] -> Compare To LKA_Min_Speed/1
  Compare To LKA_Min_Speed/1 -> Logical Operator1/5, Logical Operator2/2
  Logical Operator/1 -> Logical Operator1/4
  Logical Operator2/1 -> Data Type Conversion1/1
  Data Type Conversion1/1 -> [LKA_White]
  Demux/1 -> Logical Operator/1
  Demux/2 -> Logical Operator/2
  LKA_Lane_Gap_Activate/1(Out1) -> Logical Operator3/2, Demux/1
  Data Type Conversion3/1 -> Demux1/1
  Logical Operator3/1 -> Data Type Conversion3/1
  Rate Transition/1 -> Demux3/1, Sum of Elements/1, Discrete Derivative/1, Rate Transition1/1
  Discrete Derivative/1 -> Abs/1
  Rate Transition1/1 -> LKA_Lane_Gap_Activate/1(In1)
  Rate Transition2/1 -> Compare To LKA_Lane_Gap_dydt_Activate/1
  Compare To LKA_Lane_Gap_dydt_Activate/1 -> Demux2/1
  Logical Operator4/1 -> Logical Operator1/3
  Demux2/1 -> Logical Operator4/1
  Demux2/2 -> Logical Operator4/2
  Abs/1 -> Rate Transition2/1
  Data Type Conversion/1 -> Switch1/1, Switch1/2
  Product/1 -> Switch1/3
  Memory/1 -> Product/5
  Logical Operator5/1 -> Rate Transition5/1  "off"
  Sum of Elements/1 -> Gain1/1
  Gain1/1 -> Subtract/2  "(a+b)/2"
  Demux3/2 -> Terminator/1
  Demux3/1 -> Subtract/1
  Subtract/1 -> Saturation/1  "error from center"
  Clock/1 -> Subsystem/1(Clock)
  Compare To Constant/1 -> Logical Operator5/1  "latch_speed_off"
  Compare To Constant2/1 -> Logical Operator5/2  "latch_distance_off"
  Rate Transition5/1 -> Product/1  "toggle"
  Gain/1 -> Rate Limiter Dynamic/3
  Rate Limiter Dynamic/1 -> Product1/1
  Rate Limiter/1 -> Rate Transition3/1
  LKA_Dyn_Rate_Limiter_Power/1 -> Math Function1/2
  Math Function1/1 -> MATLAB Function/1(u)
  LKA_Dyn_Rate_Limiter_Gain/1 -> Math Function1/1
  Reciprocal/1 -> Rate Limiter Dynamic/1, Gain/1
  Abs1/1 -> Compare To Constant/1
  Discrete Derivative2/1 -> Abs2/1
  Abs2/1 -> LKA_Dyn_Rate_Limiter_Gain/1
  Abs3/1 -> Compare To Constant2/1
  Saturation/1 -> Abs3/1, Discrete Derivative1/1, [LKA_Error]
  Product1/1 -> Rate Limiter/1
  Rate Transition6/1 -> Product1/2
  Discrete Derivative1/1 -> Abs1/1, [LKA_Error_dydt]
  Pulse Generator/1 -> Product2/2
  Rate Transition3/1 -> Discrete Filter/1, Subsystem/2(Input_Signal)
  Mux3/1 -> Rate Transition/1
  [AP_On] -> Memory2/1
  Compare To Constant3/1 -> Logical Operator1/6, Logical Operator6/2
  Memory2/1 -> Compare To Constant3/1
  [Indicator_On] -> Compare To Constant4/1
  Compare To Constant4/1 -> Product/4, Logical Operator1/7, Logical Operator6/1
  Data Type Conversion2/1 -> [LKA_Ready]
  Logical Operator6/1 -> Data Type Conversion2/1
  [ADAS_Error] -> Compare To Zero/1
  Compare To Zero/1 -> Product3/1
  Product3/1 -> Logical Operator2/1, Logical Operator1/1, Product/2
  Rate Transition4/1 -> Discrete PID Controller/2(In2)
  Discrete PID Controller/1(Out1) -> Rate Limiter Dynamic/2
  Switch1/1 -> Rate Transition6/1, [LKA_Steer_Mode], [LKA_On], Sum/1, Product2/1, Rate Transition4/1, Memory/1  "LKA_on"
  [AEB_Output_Active] -> Sum/2
  Product2/1 -> [LKA_On_Pulse]
  Demux1/1 -> [LKA_On_Left]
  Demux1/2 -> [LKA_On_Right]
  Sum/1 -> [LKA_AEB_Sound]
  [LaneGap_right_ws] -> Mux3/2
  [LaneGap_left_ws] -> Mux3/1
  [LKA_White] -> Logical Operator6/3
  [LKA_Error_dydt] -> Discrete Derivative2/1
  [LKA_Error] -> Discrete PID Controller/1(In1)
  Constant1/1 -> Goto/1
  Discrete Filter/1 -> [LKA_Steer_Angle]
  LKA_Activity_Flag/1 -> Product3/2
  [LSS_controls_Start_signal] -> Product3/3
  Constant/1 -> [AEB_Output_Active], [Indicator_On], [AP_On], [ADAS_Error]
  [LKA_Steer_Angle] -> Mux/1
  [LKA_On_Pulse] -> Mux/2
  [LKA_AEB_Sound] -> Mux/3
  [LKA_On] -> Mux/4
  [LKA_Steer_Mode] -> Mux/5
  [LKA_On_Right] -> Mux/6
  [LKA_On_Left] -> Mux/7
  [LKA_Ready] -> Mux/8
  Mux/1 -> Terminator1/1
  MATLAB Function/1(y) -> Reciprocal/1

== system lss_online/OUTPUT ==
  VI-CarRealTime_Outputs : Subsystem
  WorldSim_Sensor_Outputs : Subsystem
  rough data reporting : Subsystem

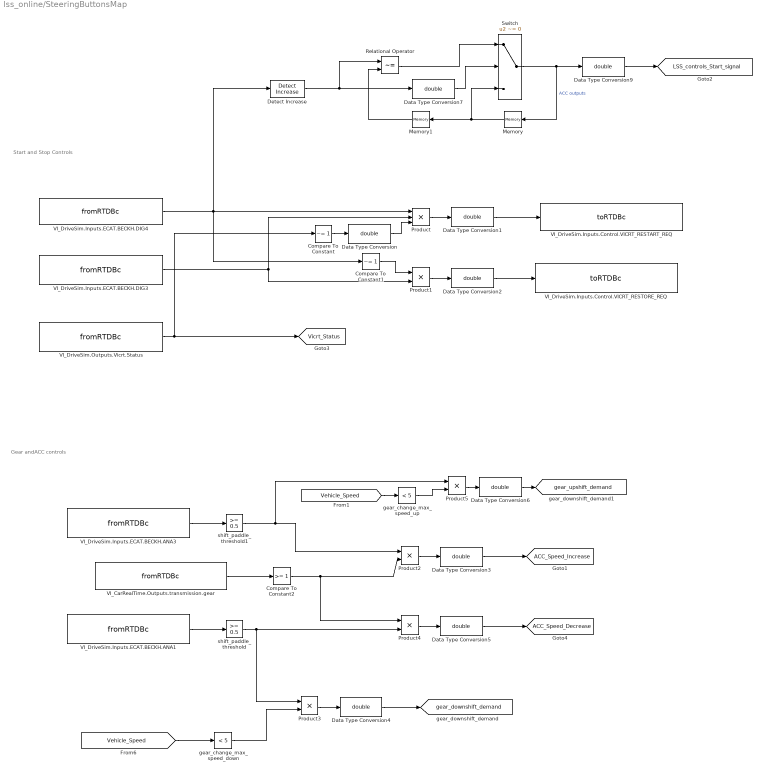
== system lss_online/SteeringButtonsMap ==
  note: Start and Stop Controls
  note: Gear andACC controls
  Compare To Constant : simulink/Logic and Bit Operations/Compare To Constant  relop=~=  const=1  OutDataTypeStr=boolean
  Compare To Constant1 : simulink/Logic and Bit Operations/Compare To Constant  relop=~=  const=1  OutDataTypeStr=boolean
  Compare To Constant2 : simulink/Logic and Bit Operations/Compare To Constant  relop=>=  const=1  OutDataTypeStr=uint8
  Data Type Conversion{,1..7,9} (9 alike) : DataTypeConversion  OutDataTypeStr=double  SaturateOnIntegerOverflow=off  RndMeth=Floor
  Detect Increase : simulink/Logic and Bit Operations/Detect Increase  vinit=0.0  InputProcessing=Columns as channels (frame based)  OutDataTypeStr=uint8
  Memory : Memory
  Memory1 : Memory
  Product : Product  Inputs=3
  Product{1..5} (5 alike) : Product
  Relational Operator : RelationalOperator  Operator=~=  OutDataTypeStr=boolean  RndMeth=Simplest  InputSameDT=off
  Switch : Switch  Criteria=u2 ~= 0  SaturateOnIntegerOverflow=off  InputSameDT=off
  VI_CarRealTime.Outputs.transmission.gear : simwbSfunlib/fromRTDBc  stringBlock=off  varName=VI_CarRealTime.Outputs.transmission.gear  sigDim=[1 1]  sigType=double  sampleTime=[-1 0]  maxBuffSize=1024  busName=nobus  defaultValue=0  defaultString=simwbin  hasMapping=0  ptrName=VI_CarRealTime_Outputs_transmission_gear  enumOrAlias=nothing
      settings: SourceProductName=SimWB MLToolkit
  VI_DriveSim.Inputs.Control.VICRT_RESTART_REQ : simwbSfunlib/toRTDBc  stringBlock=off  varName=VI_DriveSim.Inputs.Control.VICRT_RESTART_REQ  sigDim=[1 1]  sigType=double  sampleTime=[-1 0]  maxBuffSize=1024  busName=nobus  defaultValue=0  defaultString=simwbout  hasMapping=0  ptrName=VI_DriveSim_Inputs_Control_VICRT_RESTART_REQ  enumOrAlias=nothing
      settings: SourceProductName=SimWB MLToolkit
  VI_DriveSim.Inputs.Control.VICRT_RESTORE_REQ : simwbSfunlib/toRTDBc  stringBlock=off  varName=VI_DriveSim.Inputs.Control.VICRT_RESTORE_REQ  sigDim=[1 1]  sigType=double  sampleTime=[-1 0]  maxBuffSize=1024  busName=nobus  defaultValue=0  defaultString=simwbout  hasMapping=0  ptrName=VI_DriveSim_Inputs_Control_VICRT_RESTORE_REQ  enumOrAlias=nothing
      settings: SourceProductName=SimWB MLToolkit
  VI_DriveSim.Inputs.ECAT.BECKH.ANA1 : simwbSfunlib/fromRTDBc  stringBlock=off  varName=VI_DriveSim.Inputs.ECAT.BECKH.ANA4  sigDim=[1 1]  sigType=double  sampleTime=[-1 0]  maxBuffSize=1024  busName=nobus  defaultValue=0  defaultString=simwbin  hasMapping=0  ptrName=VI_DriveSim_Inputs_ECAT_BECKH_ANA4  enumOrAlias=nothing
      settings: SourceProductName=SimWB MLToolkit
  VI_DriveSim.Inputs.ECAT.BECKH.ANA3 : simwbSfunlib/fromRTDBc  stringBlock=off  varName=VI_DriveSim.Inputs.ECAT.BECKH.ANA3  sigDim=[1 1]  sigType=double  sampleTime=[-1 0]  maxBuffSize=1024  busName=nobus  defaultValue=0  defaultString=simwbin  hasMapping=0  ptrName=VI_DriveSim_Inputs_ECAT_BECKH_ANA3  enumOrAlias=nothing
      settings: SourceProductName=SimWB MLToolkit
  VI_DriveSim.Inputs.ECAT.BECKH.DIG3 : simwbSfunlib/fromRTDBc  stringBlock=off  varName=VI_DriveSim.Inputs.ECAT.BECKH.DIG3  sigDim=[1 1]  sigType=double  sampleTime=[-1 0]  maxBuffSize=1024  busName=nobus  defaultValue=0  defaultString=simwbin  hasMapping=0  ptrName=VI_DriveSim_Inputs_ECAT_BECKH_DIG3  enumOrAlias=nothing
      settings: SourceProductName=SimWB MLToolkit
  VI_DriveSim.Inputs.ECAT.BECKH.DIG4 : simwbSfunlib/fromRTDBc  stringBlock=off  varName=VI_DriveSim.Inputs.ECAT.BECKH.DIG4  sigDim=[1 1]  sigType=double  sampleTime=[-1 0]  maxBuffSize=1024  busName=nobus  defaultValue=0  defaultString=simwbin  hasMapping=0  ptrName=VI_DriveSim_Inputs_ECAT_BECKH_DIG4  enumOrAlias=nothing
      settings: SourceProductName=SimWB MLToolkit
  VI_DriveSim.Outputs.Vicrt.Status : simwbSfunlib/fromRTDBc  stringBlock=off  varName=VI_DriveSim.Outputs.Vicrt.Status  sigDim=[1 1]  sigType=double  sampleTime=[-1 0]  maxBuffSize=1024  busName=nobus  defaultValue=0  defaultString=simwbin  hasMapping=0  ptrName=VI_DriveSim_Outputs_Vicrt_Status  enumOrAlias=nothing
      settings: SourceProductName=SimWB MLToolkit
  gear_change_max_speed_down : simulink/Logic and Bit Operations/Compare To Constant  relop=<  const=5  OutDataTypeStr=uint8
  gear_change_max_speed_up : simulink/Logic and Bit Operations/Compare To Constant  relop=<  const=5  OutDataTypeStr=uint8
  shift_paddle_threshold : simulink/Logic and Bit Operations/Compare To Constant  relop=>=  const=0.5  OutDataTypeStr=uint8
  shift_paddle_threshold1 : simulink/Logic and Bit Operations/Compare To Constant  relop=>=  const=0.5  OutDataTypeStr=uint8
  tag scope: ACC_Speed_Decrease=global, ACC_Speed_Increase=global, LSS_controls_Start_signal=global, Vicrt_Status=global, gear_downshift_demand=global, gear_upshift_demand=global
  wires:
  VI_DriveSim.Inputs.ECAT.BECKH.DIG4/1 -> Detect Increase/1, Compare To Constant1/1, Product/1
  Product/1 -> Data Type Conversion1/1
  VI_DriveSim.Outputs.Vicrt.Status/1 -> [Vicrt_Status], Compare To Constant/1
  Compare To Constant/1 -> Data Type Conversion/1
  Data Type Conversion/1 -> Product/3
  VI_DriveSim.Inputs.ECAT.BECKH.DIG3/1 -> Product1/2, Product/2
  Compare To Constant1/1 -> Product1/1
  Product1/1 -> Data Type Conversion2/1
  VI_DriveSim.Inputs.ECAT.BECKH.ANA3/1 -> shift_paddle_threshold1/1
  VI_CarRealTime.Outputs.transmission.gear/1 -> Compare To Constant2/1
  Data Type Conversion1/1 -> VI_DriveSim.Inputs.Control.VICRT_RESTART_REQ/1
  Data Type Conversion2/1 -> VI_DriveSim.Inputs.Control.VICRT_RESTORE_REQ/1
  Product2/1 -> Data Type Conversion3/1
  Data Type Conversion3/1 -> [ACC_Speed_Increase]
  Compare To Constant2/1 -> Product4/1, Product2/2
  [Vehicle_Speed] -> gear_change_max_speed_down/1
  Product3/1 -> Data Type Conversion4/1
  Data Type Conversion4/1 -> [gear_downshift_demand]
  gear_change_max_speed_down/1 -> Product3/2
  Data Type Conversion5/1 -> [ACC_Speed_Decrease]
  Product4/1 -> Data Type Conversion5/1
  VI_DriveSim.Inputs.ECAT.BECKH.ANA1/1 -> shift_paddle_threshold/1
  shift_paddle_threshold/1 -> Product3/1, Product4/2
  shift_paddle_threshold1/1 -> Product5/1, Product2/1
  [Vehicle_Speed] -> gear_change_max_speed_up/1
  gear_change_max_speed_up/1 -> Product5/2
  Data Type Conversion6/1 -> [gear_upshift_demand]
  Product5/1 -> Data Type Conversion6/1
  Switch/1 -> Memory/1, Data Type Conversion9/1  "ACC outputs"
  Memory/1 -> Switch/3, Memory1/1
  Data Type Conversion9/1 -> [LSS_controls_Start_signal]
  Relational Operator/1 -> Switch/1
  Memory1/1 -> Relational Operator/2
  Detect Increase/1 -> Relational Operator/1, Data Type Conversion7/1
  Data Type Conversion7/1 -> Switch/2

== system lss_online/INPUT/Inputs for CRT ==
  Constant : Constant  Value=0
  Constant1 : Constant
  From1 : From  Commented=on  GotoTag=CC_clutch_demand  TagVisibility=global
  From2 : From  Commented=on  GotoTag=CC_throttle_demand  TagVisibility=global
  Goto : Goto  Commented=on  GotoTag=throttle_demand  TagVisibility=global
  Goto3 : Goto  Commented=on  GotoTag=clutch_demand  TagVisibility=global
  tag scope: brake_demand=global, gear_demand=global, steering_angle_demand=global, steering_torque_demand=global
  wires:
  Constant/1 -> [brake_demand]
  [LDW_Steering_Torque] -> [steering_torque_demand]
  [LKA_Steering_signal] -> [steering_angle_demand]
  From2/1 -> Goto3/1
  From1/1 -> Goto/1
  Constant1/1 -> [gear_demand]

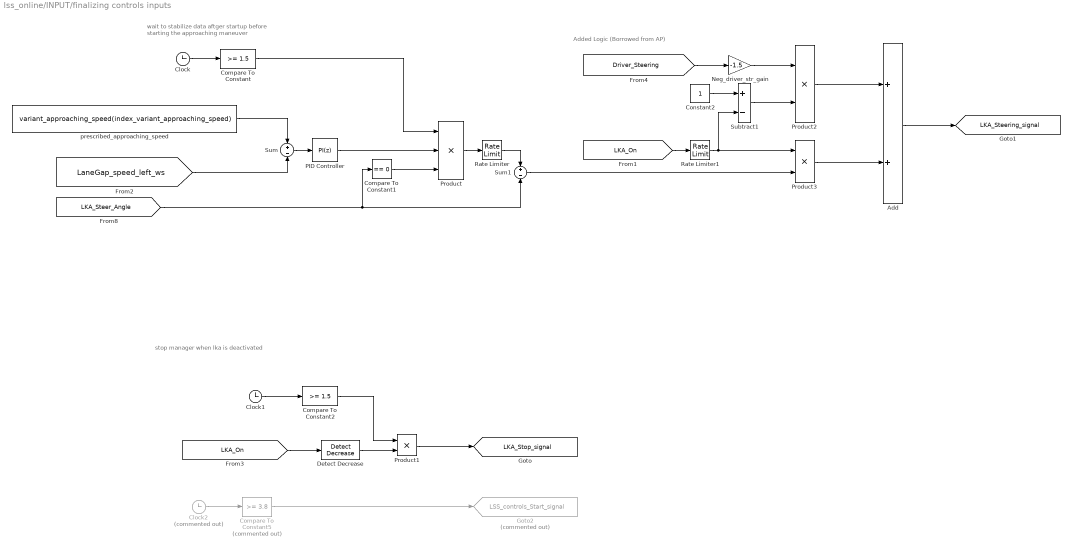
== system lss_online/INPUT/finalizing controls inputs ==
  note: Added Logic (Borrowed from AP)
  note: stop manager when lka is deactivated
  note: wait to stabilize data aftger startup
      | before starting the approaching
      | maneuver
  Add : Sum
  Clock : Clock
  Clock1 : Clock
  Clock2 : Clock  Commented=on
  Compare To Constant : simulink/Logic and Bit Operations/Compare To Constant  relop=>=  const=1.5  OutDataTypeStr=boolean
  Compare To Constant1 : simulink/Logic and Bit Operations/Compare To Constant  relop===  const=0  OutDataTypeStr=boolean
  Compare To Constant2 : simulink/Logic and Bit Operations/Compare To Constant  relop=>=  const=1.5  OutDataTypeStr=boolean
  Compare To Constant5 : simulink/Logic and Bit Operations/Compare To Constant  Commented=on  relop=>=  const=3.8  OutDataTypeStr=boolean
  Constant2 : Constant
  Detect Decrease : simulink/Logic and Bit Operations/Detect Decrease  vinit=0.0  OutDataTypeStr=boolean
  Goto2 : Goto  Commented=on  GotoTag=LSS_controls_Start_signal  TagVisibility=global
  Neg_driver_str_gain : Gain  Gain=-1.5
  PID Controller : slpidlib/PID Controller  Controller=PI  Form=Parallel  TimeDomain=Discrete-time  UseExternalTs=off  SampleTime=-1  IntegratorMethod=Forward Euler  FilterMethod=Forward Euler  ControllerParametersSource=internal  P=0.4  I=-0.002  UseKiTs=off  D=0  N=100  UseFilter=on  TunerSelectOption=Transfer Function Based (PID Tuner App)  InitialConditionSource=internal  InitialConditionForIntegrator=0  InitialConditionForFilter=0  DifferentiatorICPrevScaledInput=0  ExternalReset=none  TrackingMode=off  Kt=1  LimitOutput=off  SatLimitsSource=internal  UpperSaturationLimit=inf  LowerSaturationLimit=-inf  LinearizeAsGain=on  AntiWindupMode=none  Kb=1  LimitIntegrator=off  UpperIntegratorSaturationLimit=inf  LowerIntegratorSaturationLimit=-inf  POutMin=[]  POutMax=[]  IOutMin=[]  IOutMax=[]  DOutMin=[]  DOutMax=[]  NOutMin=[]  NOutMax=[]  SumOutMin=[]  SumOutMax=[]  SaturationOutMin=[]  SaturationOutMax=[]  PParamMin=[]  PParamMax=[]  IParamMin=[]  IParamMax=[]  DParamMin=[]  DParamMax=[]  NParamMin=[]  NParamMax=[]  KbParamMin=[]  KbParamMax=[]  KtParamMin=[]  KtParamMax=[]  KbOutMin=[]  KbOutMax=[]  KtOutMin=[]  KtOutMax=[]  IntegratorOutMin=[]  IntegratorOutMax=[]  FilterOutMin=[]  FilterOutMax=[]  SumI1OutMin=[]  SumI1OutMax=[]  SumI2OutMin=[]  SumI2OutMax=[]  SumI3OutMin=[]  SumI3OutMax=[]  SumI4OutMin=[]  SumI4OutMax=[]  SumDOutMin=[]  SumDOutMax=[]  DifferentiatorOutMin=[]  DifferentiatorOutMax=[]  FilterDiffOutCoefMin=[]  FilterDiffOutCoefMax=[]  ReciprocalOutMin=[]  ReciprocalOutMax=[]  SumDenOutMin=[]  SumDenOutMax=[]  SumNumOutMin=[]  SumNumOutMax=[]  DivideOutMin=[]  DivideOutMax=[]  UdiffTsProdOutMin=[]  UdiffTsProdOutMax=[]  NTsProdOutMin=[]  NTsProdOutMax=[]  UintegralTsProdOutMin=[]  UintegralTsProdOutMax=[]  UngainTsProdOutMin=[]  UngainTsProdOutMax=[]  ClampingZeroOutDataTypeStr=Inherit: Inherit via back propagation  ClampingZeroOutMin=[]  ClampingZeroOutMax=[]  FilterDenConstantOutDataTypeStr=Inherit: Inherit via back propagation  FilterDenConstantOutMin=[]  FilterDenConstantOutMax=[]  PCopyOutDataTypeStr=Inherit: Inherit via back propagation  PCopyOutMin=[]  PCopyOutMax=[]  NCopyOutDataTypeStr=Inherit: Inherit via back propagation  NCopyOutMin=[]  NCopyOutMax=[]  IntegratorContinuousStateAttributes=''  IntegratorStateMustResolveToSignalObject=off  IntegratorRTWStateStorageClass=Auto  FilterContinuousStateAttributes=''  FilterStateMustResolveToSignalObject=off  FilterRTWStateStorageClass=Auto  ParallelPVariant=InternalParameters  IdealPVariant=Disabled  IVariant=InternalParameters  DVariant=Disabled  IntegratorVariant=Discrete  SatVariant=Disabled  AWVariant=Passthrough  PCopyVariant=Disabled  TRVariant=Disabled  FdbkBlocksVariant=Forward  IdealPFdbkVariant=Disabled  SatFdbkVariant=Disabled  DerivativeFilterVariant=Disabled  NVariant=Disabled  NCopyVariant=Disabled_SignalSpec  FilterICVariant=Disabled  IntegratorICVariant=InternalICs  ExternalResetVariant=Disabled  TRSumVariant=Passthrough  SumFdbkVariant=Disabled  SumVariant=Sum_PI  TsampFilterVariant=InternalTs  TsampNgainVariant=Passthrough  TsampIntegralVariant=Passthrough  ExternalSaturationOutDataTypeStr=Inherit: Same as second input
  Product : Product  Inputs=3
  Product1 : Product
  Product2 : Product
  Product3 : Product
  Rate Limiter : RateLimiter  RisingSlewLimit=0.75  FallingSlewLimit=-inf  SampleTimeMode=inherited
  Rate Limiter1 : RateLimiter  RisingSlewLimit=AP_Transition_Rate  FallingSlewLimit=-AP_Transition_Rate  SampleTimeMode=inherited
  Subtract1 : Sum  Inputs=+-
  Sum : Sum  Inputs=+-
  Sum1 : Sum  Inputs=+-
  prescribed_approaching_speed : Constant  Value=variant_approaching_speed(index_variant_approaching_speed)
  tag scope: LKA_Steering_signal=global, LKA_Stop_signal=global
  wires:
  Compare To Constant2/1 -> Product1/1
  [LaneGap_speed_left_ws] -> Sum/2
  Clock/1 -> Compare To Constant/1
  [LKA_Steer_Angle] -> Compare To Constant1/1, Sum1/2
  Product/1 -> Rate Limiter/1
  prescribed_approaching_speed/1 -> Sum/1
  Sum/1 -> PID Controller/1
  Compare To Constant1/1 -> Product/3
  Detect Decrease/1 -> Product1/2
  Compare To Constant/1 -> Product/1
  Product1/1 -> [LKA_Stop_signal]
  PID Controller/1 -> Product/2
  Clock1/1 -> Compare To Constant2/1
  [LKA_On] -> Detect Decrease/1
  Compare To Constant5/1 -> Goto2/1
  Clock2/1 -> Compare To Constant5/1
  Rate Limiter/1 -> Sum1/1
  [Driver_Steering] -> Neg_driver_str_gain/1
  Add/1 -> [LKA_Steering_signal]
  [LKA_On] -> Rate Limiter1/1
  Sum1/1 -> Product3/2
  Constant2/1 -> Subtract1/1
  Product3/1 -> Add/2
  Product2/1 -> Add/1
  Rate Limiter1/1 -> Subtract1/2, Product3/1
  Subtract1/1 -> Product2/2
  Neg_driver_str_gain/1 -> Product2/1
